simulink model "protocol"  (R2021b)
settings: Solver=VariableStepAuto  StartTime=0.0  StopTime=10.0  RelTol=1e-3
settings Model: Creator=marco  LastModifiedBy=marco

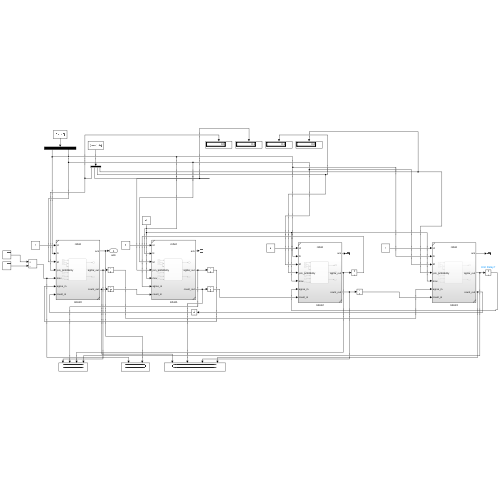
[thumbnail: Simulink's stored preview of the top-level diagram]
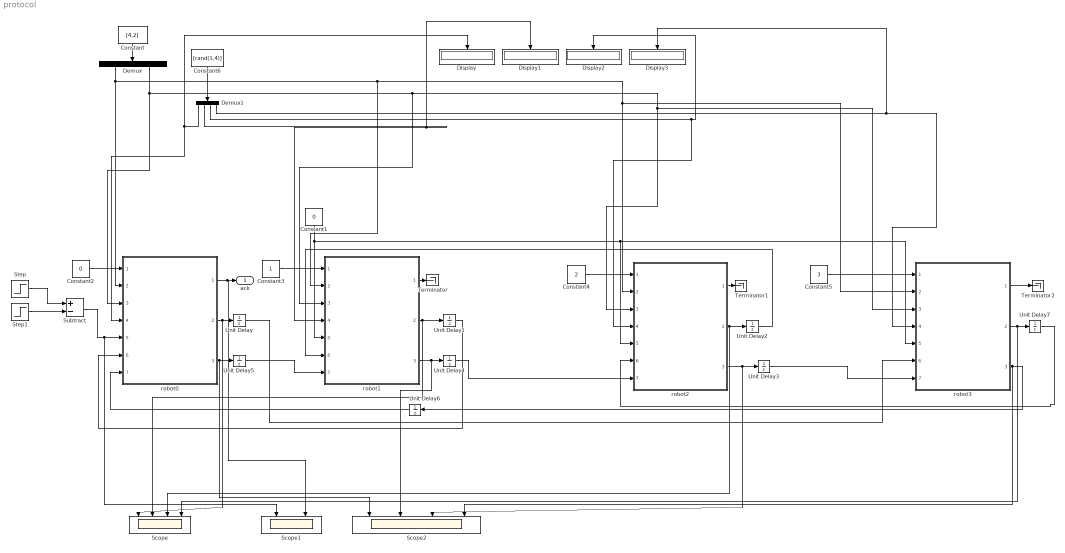
== system protocol ==
  Constant : Constant  Value=[4,2]
  Constant1 : Constant  Value=0
  Constant2 : Constant  Value=0
  Constant3 : Constant
  Constant4 : Constant  Value=2
  Constant5 : Constant  Value=3
  Constant6 : Constant  Value=[rand(1,4)]
  Demux : Demux  Outputs=2
  Demux1 : Demux
  Display{,1..3} (4 alike) : Display
  Scope : Scope  NumInputPorts=4
  Scope1 : Scope  NumInputPorts=2
  Scope2 : Scope  NumInputPorts=4
  Step : Step  SampleTime=.2
  Step1 : Step  Time=1.2  SampleTime=.2
  Subtract : Sum  Inputs=+-
  Terminator : Terminator
  Terminator1 : Terminator
  Terminator2 : Terminator
  Unit Delay{,1..7} (8 alike) : UnitDelay  SampleTime=-1  HasFrameUpgradeWarning=on
  robot{0..3} (4 alike) : Subsystem  ReferencedSubsystem=robot
  ack : Outport
  wires:
  Demux/1 -> robot0/2, robot1/2, robot3/2, robot2/2
  Demux/2 -> robot0/3, robot1/3, robot3/3, robot2/3
  Demux1/1 -> robot0/4, Display/1
  Constant/1 -> Demux/1
  Constant6/1 -> Demux1/1
  Demux1/2 -> robot1/4, Display1/1
  Demux1/3 -> robot2/4, Display2/1
  Demux1/4 -> robot3/4, Display3/1
  robot3/2 -> Scope/4, Unit Delay7/1
  robot0/2 -> Scope/1, Unit Delay/1
  robot1/2 -> Scope/2, Unit Delay1/1
  robot2/2 -> Scope/3, Unit Delay2/1
  robot0/3 -> Scope2/1, Unit Delay5/1
  robot1/3 -> Scope2/2, Unit Delay4/1
  robot2/3 -> Scope2/3, Unit Delay3/1
  robot3/3 -> Unit Delay6/1, Scope2/4
  Unit Delay3/1 -> robot3/7
  Unit Delay4/1 -> robot2/7
  Unit Delay5/1 -> robot1/7
  Unit Delay6/1 -> robot0/7
  Unit Delay1/1 -> robot0/6
  robot0/1 -> Scope1/2, ack/1
  robot1/1 -> Terminator/1
  robot2/1 -> Terminator1/1
  robot3/1 -> Terminator2/1
  Constant1/1 -> robot3/5, robot2/5, robot1/5
  Constant2/1 -> robot0/1
  Constant3/1 -> robot1/1
  Constant4/1 -> robot2/1
  Constant5/1 -> robot3/1
  Step/1 -> Subtract/1
  Step1/1 -> Subtract/2
  Subtract/1 -> Scope1/1, robot0/5
  Unit Delay2/1 -> robot1/6
  Unit Delay7/1 -> robot2/6
  Unit Delay/1 -> robot3/6
